simulink model "data"  (R2020a)
settings: Solver=VariableStepAuto  StartTime=0.0  StopTime=10.0  RelTol=1e-3
undefined symbols (not defined in the file): A, B, C
settings Model: DataDictionary=datadict.sldd  Creator=NIKITA  LastModifiedBy=NIKITA

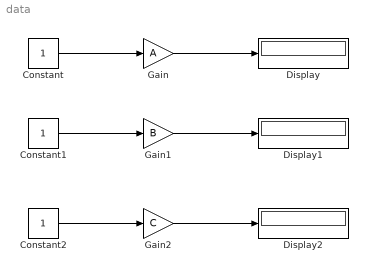
== system data ==
  Constant : Constant
  Constant1 : Constant
  Constant2 : Constant
  Display : Display
  Display1 : Display
  Display2 : Display
  Gain : Gain  Gain=A
  Gain1 : Gain  Gain=B
  Gain2 : Gain  Gain=C
  wires:
  Constant2/1 -> Gain2/1
  Constant1/1 -> Gain1/1
  Constant/1 -> Gain/1
  Gain2/1 -> Display2/1
  Gain1/1 -> Display1/1
  Gain/1 -> Display/1
